simulink model "Regular_Drone"  (R2022b)
settings: Solver=VariableStepAuto  StartTime=0.0  StopTime=5  RelTol=1e-3
model workspace (MAT data in the model file):
  test = [0.0018504  0  0; 0  0.0018507  0; 0  0  0.0029763]
undefined symbols (not defined in the file): Od, omegad, pd, vd
libraries: robotgazebolib x5
settings Model: Creator=Daniel Angkiat  LastModifiedBy=daniel

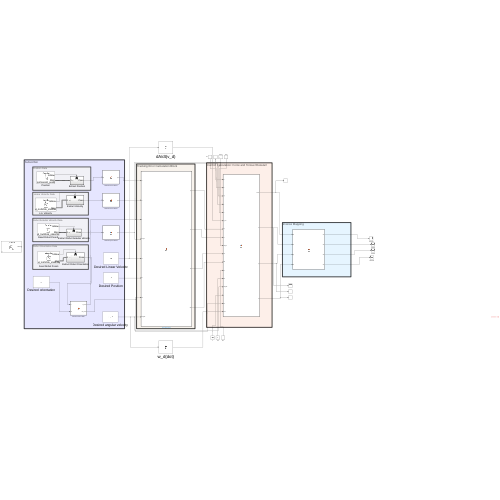
[thumbnail: Simulink's stored preview of the top-level diagram]
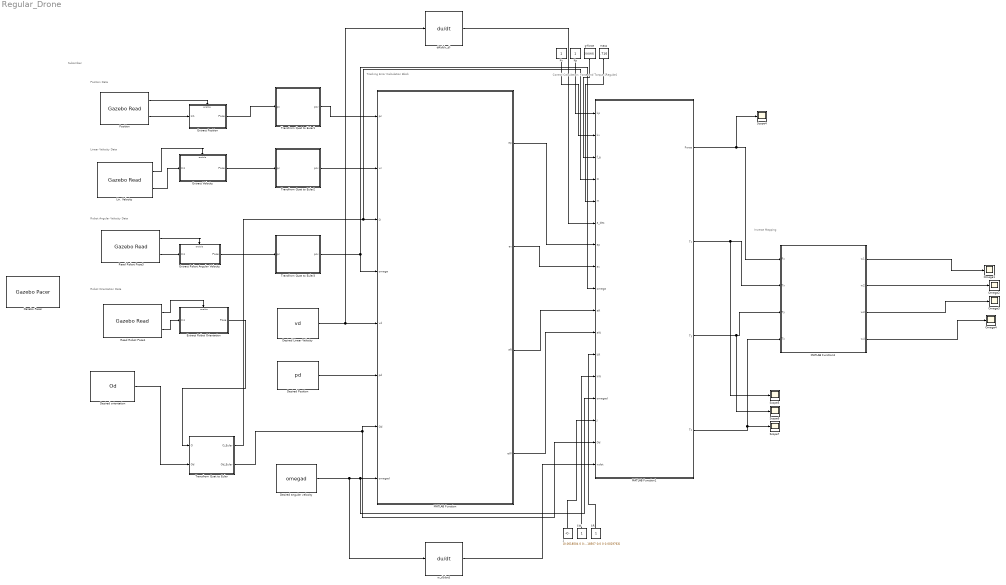
== system Regular_Drone ==
  note: Subscriber
  note: Robot Orientation Data
  note: Linear Velocity Data
  note: Robot Angular Velocity Data
  note: Position Data
  note: Tracking Error Calculation Block
  note: Control Calculation; Force and Torque [Regular]
  note: Inverse Mapping
  Desired Linear Velocity : Constant  Value=vd  VectorParams1D=off
  Desired Position : Constant  Value=pd  VectorParams1D=off
  Desired angular velocity : Constant  Value=omegad  VectorParams1D=off
  Desired orientation : Constant  Value=Od  VectorParams1D=off
  Extract Position : Subsystem
  Extract Robot Angular Velocity : Subsystem
  Extract Robot Orientation : Subsystem
  Extract Velocity : Subsystem
  Gazebo Pacer : robotgazebolib/Gazebo Pacer  ResetBehavior=Reset Gazebo simulation time  SampleTime=0.01
  J : Constant  Value=[0.0018504 0 0;0 0.0018507 0;0 0 0.0029763]  VectorParams1D=off
  Kp : Constant
  Kv : Constant
  Lin. Velocity : robotgazebolib/Gazebo Read  topicSource=From Gazebo  topic=/gazebo/ground_truth/link_state/test10/base_link  messageType=gazebo_msgs/LinkState  sampleTime=0.01  fixedAxisBusStatus=off  jointAxisCount=2
  MATLAB Function : MATLAB Function  TreatAsAtomicUnit=on
  MATLAB Function1 : MATLAB Function  TreatAsAtomicUnit=on
  MATLAB Function3 : MATLAB Function  TreatAsAtomicUnit=on
  Omega{1..4} (4 alike) : Scope
  Position : robotgazebolib/Gazebo Read  topicSource=From Gazebo  topic=/gazebo/ground_truth/world_pose/test10/base_link  messageType=gazebo_msgs/Pose  sampleTime=0.01  fixedAxisBusStatus=off  jointAxisCount=2
  Read Robot Pose1 : robotgazebolib/Gazebo Read  topicSource=From Gazebo  topic=/gazebo/ground_truth/link_state/test10/base_link  messageType=gazebo_msgs/LinkState  sampleTime=0.01  fixedAxisBusStatus=off  jointAxisCount=2
  Read Robot Pose3 : robotgazebolib/Gazebo Read  topicSource=From Gazebo  topic=/gazebo/ground_truth/link_state/test10/base_link  messageType=gazebo_msgs/LinkState  sampleTime=0.01  fixedAxisBusStatus=off  jointAxisCount=2
  Scope{4..7} (4 alike) : Scope
  Transfrom Quat to Euler : MATLAB Function  TreatAsAtomicUnit=on
  Transfrom Quat to Euler1 : MATLAB Function  TreatAsAtomicUnit=on
  Transfrom Quat to Euler2 : MATLAB Function  TreatAsAtomicUnit=on
  Transfrom Quat to Euler3 : MATLAB Function  TreatAsAtomicUnit=on
  dA/dt(v_d) : Derivative
  g-force : Constant  Value=[0;0;9.8]  VectorParams1D=off
  kR : Constant
  kW : Constant
  mass : Constant  Value=.716
  "w_d{dot}" : Derivative
  wires:
  Position/1 -> Extract Position/Enable
  Read Robot Pose1/2 -> Extract Robot Orientation/1(In1)
  Read Robot Pose1/1 -> Extract Robot Orientation/Enable
  Lin. Velocity/1 -> Extract Velocity/Enable
  Read Robot Pose3/1 -> Extract Robot Angular Velocity/Enable
  Position/2 -> Extract Position/1(In1)
  Read Robot Pose3/2 -> Extract Robot Angular Velocity/1(In1)
  Lin. Velocity/2 -> Extract Velocity/1(In1)
  Extract Position/1(Pose) -> Transfrom Quat to Euler1/1(pc)
  Desired Position/1 -> MATLAB Function/6(pd)
  Desired Linear Velocity/1 -> dA/dt(v_d)/1, MATLAB Function/5(vd)
  Desired angular velocity/1 -> "w_d{dot}"/1, MATLAB Function1/14(omegad), MATLAB Function/8(omegad)
  MATLAB Function/1(ep) -> MATLAB Function1/7(ep)
  MATLAB Function/2(ev) -> MATLAB Function1/8(ev)
  dA/dt(v_d)/1 -> MATLAB Function1/6(a_des)
  Kp/1 -> MATLAB Function1/1(kp)
  Kv/1 -> MATLAB Function1/2(kv)
  g-force/1 -> MATLAB Function1/3(f_g)
  mass/1 -> MATLAB Function1/5(m)
  "w_d{dot}"/1 -> MATLAB Function1/17(wdot)
  J/1 -> MATLAB Function1/15(J)
  kR/1 -> MATLAB Function1/12(kR)
  kW/1 -> MATLAB Function1/13(kW)
  MATLAB Function/3(eR) -> MATLAB Function1/10(eR)
  MATLAB Function/4(eW) -> MATLAB Function1/11(eW)
  ? -> ?
  Extract Robot Orientation/1(Pose) -> Transfrom Quat to Euler/1(O)
  Desired orientation/1 -> Transfrom Quat to Euler/2(Od)
  Transfrom Quat to Euler/1(O_Euler) -> MATLAB Function1/4(O), MATLAB Function/3(O)
  Transfrom Quat to Euler/2(Od_Euler) -> MATLAB Function/7(Od), MATLAB Function1/16(Od)
  Transfrom Quat to Euler1/1(pcv) -> MATLAB Function/1(pc)
  Extract Velocity/1(Pose) -> Transfrom Quat to Euler2/1(pc)
  Extract Robot Angular Velocity/1(Pose) -> Transfrom Quat to Euler3/1(pc)
  Transfrom Quat to Euler2/1(pcv) -> MATLAB Function/2(vc)
  Transfrom Quat to Euler3/1(pcv) -> MATLAB Function/4(omega), MATLAB Function1/9(omega)
  MATLAB Function1/2(Tx) -> Scope5/1, MATLAB Function3/2(Tx)
  MATLAB Function1/3(Ty) -> Scope6/1, MATLAB Function3/3(Ty)
  MATLAB Function1/4(Tz) -> MATLAB Function3/4(Tz), Scope7/1
  MATLAB Function3/1(w1) -> Omega1/1
  MATLAB Function3/2(w2) -> Omega2/1
  MATLAB Function3/3(w3) -> Omega3/1
  MATLAB Function3/4(w4) -> Omega4/1
  MATLAB Function1/1(Force) -> Scope4/1, MATLAB Function3/1(Fz)

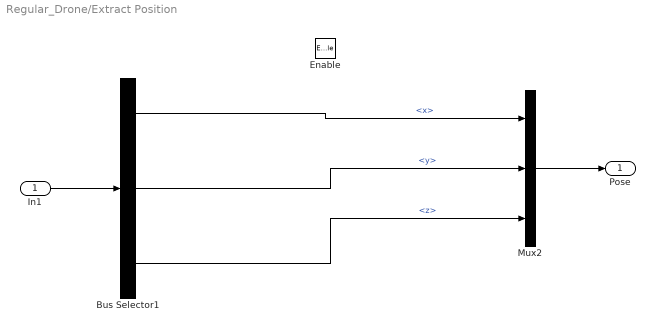
== system Regular_Drone/Extract Position ==
  In1 : Inport
  Enable : EnablePort
  Bus Selector1 : BusSelector  OutputSignals=position.x,position.y,position.z
  Mux2 : Mux  Inputs=3
  Pose : Outport  VectorParamsAs1DForOutWhenUnconnected=off
  wires:
  Mux2/1 -> Pose/1
  Bus Selector1/3 -> Mux2/3  "<z>"
  In1/1 -> Bus Selector1/1
  Bus Selector1/2 -> Mux2/2  "<y>"
  Bus Selector1/1 -> Mux2/1  "<x>"

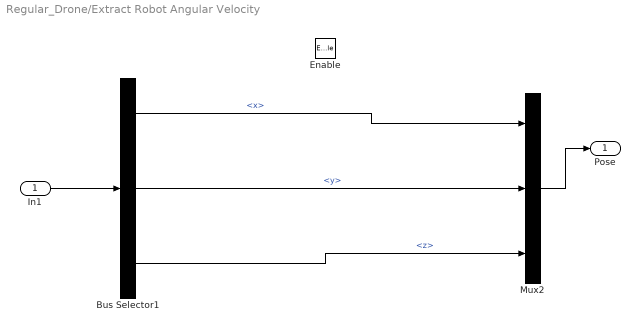
== system Regular_Drone/Extract Robot Angular Velocity ==
  In1 : Inport
  Enable : EnablePort
  Bus Selector1 : BusSelector  OutputSignals=relative_angular_velocity.x,relative_angular_velocity.y,relative_angular_velocity.z
  Mux2 : Mux  Inputs=3
  Pose : Outport  VectorParamsAs1DForOutWhenUnconnected=off
  wires:
  Mux2/1 -> Pose/1
  Bus Selector1/1 -> Mux2/1  "<x>"
  In1/1 -> Bus Selector1/1
  Bus Selector1/3 -> Mux2/3  "<z>"
  Bus Selector1/2 -> Mux2/2  "<y>"

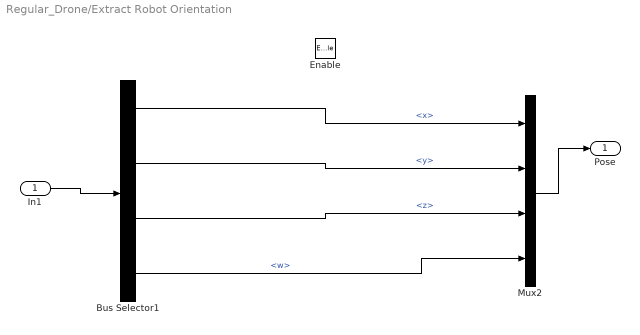
== system Regular_Drone/Extract Robot Orientation ==
  In1 : Inport
  Enable : EnablePort
  Bus Selector1 : BusSelector  OutputSignals=world_pose.orientation.x,world_pose.orientation.y,world_pose.orientation.z,world_pose.orientation.w
  Mux2 : Mux
  Pose : Outport  VectorParamsAs1DForOutWhenUnconnected=off
  wires:
  Mux2/1 -> Pose/1
  Bus Selector1/1 -> Mux2/1  "<x>"
  In1/1 -> Bus Selector1/1
  Bus Selector1/2 -> Mux2/2  "<y>"
  Bus Selector1/3 -> Mux2/3  "<z>"
  Bus Selector1/4 -> Mux2/4  "<w>"

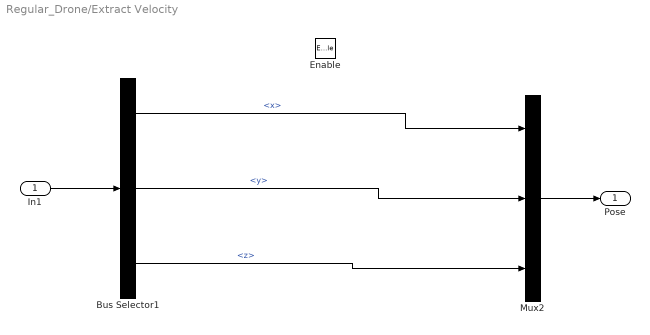
== system Regular_Drone/Extract Velocity ==
  In1 : Inport
  Enable : EnablePort
  Bus Selector1 : BusSelector  OutputSignals=world_linear_velocity.x,world_linear_velocity.y,world_linear_velocity.z
  Mux2 : Mux  Inputs=3
  Pose : Outport  VectorParamsAs1DForOutWhenUnconnected=off
  wires:
  Mux2/1 -> Pose/1
  Bus Selector1/1 -> Mux2/1  "<x>"
  In1/1 -> Bus Selector1/1
  Bus Selector1/2 -> Mux2/2  "<y>"
  Bus Selector1/3 -> Mux2/3  "<z>"

== matlab function Regular_Drone/MATLAB Function1 ==
  data: kp input; kv input; f_g input; O input; m input; a_des input; Force output; ep input; ev input; omega input; eR input; eW input; Tx output; kR input; kW input; omegad input; J input; Od input; wdot input; Ty output; Tz output
function [Force,Tx,Ty,Tz] = fcn(kp,kv,f_g,O,m,a_des,ep,ev,omega,eR,eW,kR,kW,omegad,J,Od,wdot)

% Force

e3 = [0;0;1]; % Z-Directional Force 
temp = -O'*e3;
F = (-kp*ep-kv*ev-f_g+m*a_des)*temp;
Force = F(3);
% Torque
Torque = -kR*eR-kW*eW+cross(J*omega,omega)
% lol = cross(J*omega, omega);
% tempvar1 = (-kR.*eR-kW.*eW+lol);
% tempvar2 = O'*Od*omegad; 
% tempvar3 = O'*Od*wdot;
% Torque = tempvar1 - J*(cross(omega,tempvar2)-tempvar3);
Tx = Torque(1);
Ty = Torque(2);
Tz = Torque(3);

== matlab function Regular_Drone/MATLAB Function ==
  data: pc input; vc input; O input; omega input; vd input; ep output; ev output; eR output; pd input; Od input; omegad input; eW output
function [ep, ev, eR, eW] = fcn(pc,vc,O,omega,vd,pd,Od,omegad)

%% Error for Position
ep = pc-pd;


%% Error for Position
ev = vc-vd;


%% Error for Orientation
tempvar = (1/2)*(Od'*O-O'*Od);
eR = tempvar; 
%[tempvar(8);tempvar(3);tempvar(4)]; % This is using the transformation of

% [0 -c b]
% [c 0 -a] ==> N; N^V = [a;b;c]   
% [-b a 0]

%% Error for Angular Velocity
tempvar2 = O'*Od*omegad;
eW = omega - tempvar2;

== matlab function Regular_Drone/Transfrom Quat to Euler ==
  data: O input; O_Euler output; Od input; Od_Euler output
function [O_Euler, Od_Euler] = fcn(O,Od)

temp1 = quat2eul([Od(1) Od(2) Od(3) Od(4)])';
Od_Euler = temp1; 
%[temp1(1) 0 0; 0 temp1(2) 0; 0 0 temp1(3)];
temp2 = quat2eul([O(1) O(2) O(3) O(4)])';
O_Euler = temp2;
% [temp2(1) 0 0; 0 temp2(2) 0; 0 0 temp2(3)];

== matlab function Regular_Drone/Transfrom Quat to Euler1 ==
  data: pc input; pcv output
function pcv  = fcn(pc)

pcv = [pc(1); pc(2); pc(3)];

== matlab function Regular_Drone/Transfrom Quat to Euler2 ==
  data: pc input; pcv output
function pcv  = fcn(pc)

pcv = [pc(1); pc(2); pc(3)];

== matlab function Regular_Drone/Transfrom Quat to Euler3 ==
  data: pc input; pcv output
function pcv  = fcn(pc)

pcv = [pc(1); pc(2); pc(3)];

== matlab function Regular_Drone/MATLAB Function3 ==
  data: Fz input; Tx input; Ty input; Tz input; w1 output; w2 output; w3 output; w4 output
function [w1, w2, w3, w4] = fcn(Fz, Tx, Ty, Tz)
cf = 1;
cd = 0.1;
g = 9.81;
d = 0.4; % Check URDF for the real value, this is only used for now
e3 = [0;0;1];
a = cf*d/sqrt(2);

F2W = [cf,cf,cf,cf;
        a,a,-a,-a;
        -a,a,a,-a;
        cd, -cd, cd,-cd];
temp = [Fz;Tx;Ty;Tz];
w_squared = F2W\temp;
w = [0, 0, 0, 0];
for i = 1:4
    if w_squared(i) < 0
        w(i) = -sqrt(-w_squared(i))
    else
        w(i) = sqrt(w_squared(i))
    end
end
w1 = w(1);
w2 = w(2);
w3 = w(3);
w4 = w(4);
